simulink model "r"  (R2014b)
settings: Solver=FixedStepDiscrete  StartTime=0.0  StopTime=sim_time_step_size  FixedStep=sim_time_step_size  RelTol=1e-3
values from neighbouring files (symbols this model uses):
  sim_time_step_size = 1/100    (= 0.01)    [nimbus_sim_init.m]
undefined symbols (not defined in the file or in its folder): ini_epoch_seconds, ini_tgt_landing_mcmf_pos
libraries: util_frame_rotation_lib x3
settings Model: Creator=Jim Kaidy  LastModifiedBy=mstewart
settings DataIOCC: SignalLoggingSaveFormat=ModelDataLogs
settings OptimizationCC: ExpressionDepthLimit=2147483647
settings DebuggingCC: UnderspecifiedInitializationDetection=Classic  MergeDetectMultiDrivingBlocksExec=none  FcnCallInpInsideContextMsg=EnableAllAsWarning  StateNameClashWarn=warning

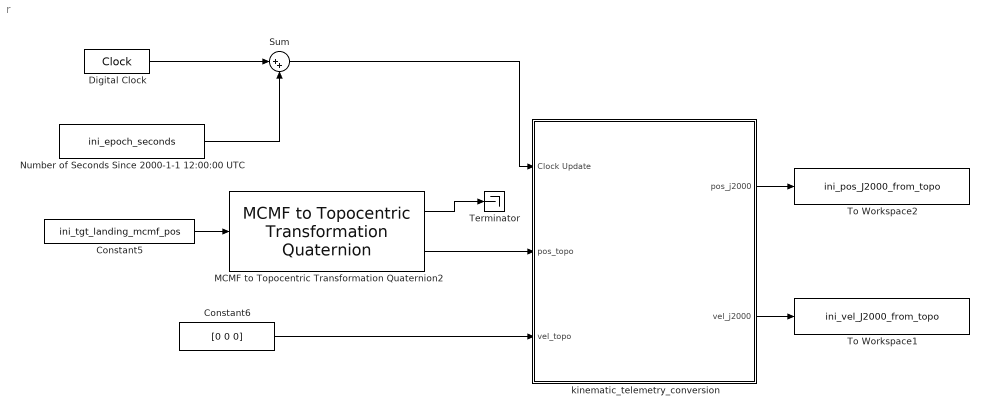
== system r ==
  Constant5 : Constant  Value=ini_tgt_landing_mcmf_pos
  Constant6 : Constant  Value=[0 0 0]
  Digital Clock : DigitalClock  SampleTime=sim_time_step_size
  MCMF to Topocentric Transformation Quaternion2 : util_frame_rotation_lib/MCMF to Topocentric  Transformation Quaternion  SystemSampleTime=-1
  Number of Seconds Since 2000-1-1 12:00:00 UTC : Constant  Description=|  Value=ini_epoch_seconds
      | Number of Seconds                   
      | July 4, 2014 22:40:00 UTC           
      | Calculate on Web Site:              
      | www.mbari.org/staff/rich/utccalc.htm
  Sum : Sum  Inputs=|++
  Terminator : Terminator
  To Workspace1 : ToWorkspace  VariableName=ini_vel_J2000_from_topo  SaveFormat=Timeseries  SampleTime=-1
  To Workspace2 : ToWorkspace  VariableName=ini_pos_J2000_from_topo  SaveFormat=Timeseries  SampleTime=-1
  kinematic_telemetry_conversion : Subsystem
  wires:
  kinematic_telemetry_conversion/2(vel_j2000) -> To Workspace1/1
  Constant6/1 -> kinematic_telemetry_conversion/3(vel_topo)
  Number of Seconds Since 2000-1-1 12:00:00 UTC/1 -> Sum/2
  Digital Clock/1 -> Sum/1
  Sum/1 -> kinematic_telemetry_conversion/1(Clock Update)
  Constant5/1 -> MCMF to Topocentric Transformation Quaternion2/1
  MCMF to Topocentric Transformation Quaternion2/2 -> kinematic_telemetry_conversion/2(pos_topo)
  MCMF to Topocentric Transformation Quaternion2/1 -> Terminator/1
  kinematic_telemetry_conversion/1(pos_j2000) -> To Workspace2/1

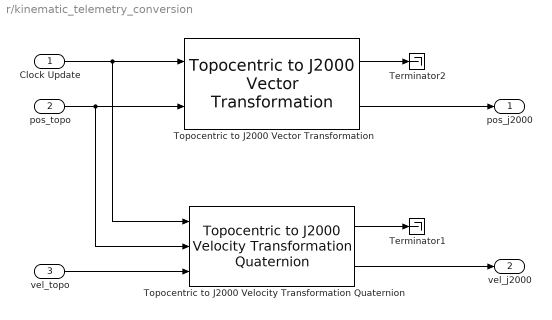
== system r/kinematic_telemetry_conversion ==
  Clock Update : Inport
  pos_topo : Inport  Port=2
  vel_topo : Inport  Port=3
  Terminator1 : Terminator
  Terminator2 : Terminator
  "Topocentric to J2000 Vector Transformation " : util_frame_rotation_lib/Topocentric to J2000 Vector Transformation   SystemSampleTime=-1
  Topocentric to J2000 Velocity Transformation Quaternion : util_frame_rotation_lib/Topocentric to J2000 Velocity  Transformation Quaternion  SystemSampleTime=-1
  pos_j2000 : Outport
  vel_j2000 : Outport  Port=2
  wires:
  Clock Update/1 -> "Topocentric to J2000 Vector Transformation "/1, Topocentric to J2000 Velocity Transformation Quaternion/1
  pos_topo/1 -> Topocentric to J2000 Velocity Transformation Quaternion/2, "Topocentric to J2000 Vector Transformation "/2
  vel_topo/1 -> Topocentric to J2000 Velocity Transformation Quaternion/3
  Topocentric to J2000 Velocity Transformation Quaternion/2 -> vel_j2000/1
  Topocentric to J2000 Velocity Transformation Quaternion/1 -> Terminator1/1
  "Topocentric to J2000 Vector Transformation "/1 -> Terminator2/1
  "Topocentric to J2000 Vector Transformation "/2 -> pos_j2000/1
